simulink model "buck1"  (Simulink 6.1)
settings: Solver=ode45  StartTime=0.0  StopTime=0.01  RelTol=1e-3
libraries: powerlib x11
settings Model: Creator=USRE  LastModifiedBy=Sreejith
settings OptimizationCC: InlineInvariantSignals=off  InitFltsAndDblsToZero=off
settings DebuggingCC: SignalResolutionControl=UseLocalSettings  SolverPrmCheckMsg=warning  MultiTaskDSMMsg=error
settings GRTTargetCC: TargetFcnLib=ansi_tfl_table_tmw.mat

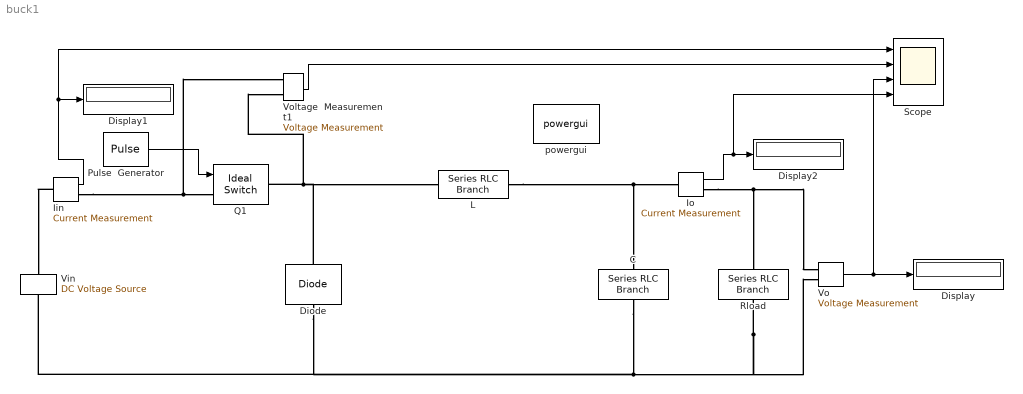
== system buck1 ==
  C : powerlib/Elements/Series RLC Branch  Orientation=down  PhysicalDomain=powersysdomain  SubClassName=unknown  LeftPortType=p1  RightPortType=p1  LConnTagsString=__new0  RConnTagsString=__new0  Resistance=0.1  Inductance=1e-3  Capacitance=120e-6  Measurements=Branch voltage
  Diode : powerlib/Power Electronics/Diode  Orientation=up  Ron=0.001  Lon=0  Vf=0.8  IC=0  Rs=500  Cs=250e-9  Measurements=off
  Display : Display
  Display1 : Display
  Display2 : Display
  Iin : powerlib/Measurements/Current Measurement  PhasorSimulation=off  OutputType=Complex  PSBequivalent=0
  Io : powerlib/Measurements/Current Measurement  PhasorSimulation=off  OutputType=Complex  PSBequivalent=0
  L : powerlib/Elements/Series RLC Branch  PhysicalDomain=powersysdomain  SubClassName=unknown  LeftPortType=p1  RightPortType=p1  LConnTagsString=__new0  RConnTagsString=__new0  Resistance=1  Inductance=11.5e-6  Capacitance=1e-6  Measurements=None
  Pulse  Generator : DiscretePulseGenerator  PulseType=Time based  Period=1/(100e3)  PulseWidth=50
  Q1 : powerlib/Power Electronics/Ideal Switch  Ron=0.001  Lon=0  IC=0  Rs=1e5  Cs=inf  Measurements=off
  Rload : powerlib/Elements/Series RLC Branch  Orientation=down  PhysicalDomain=powersysdomain  SubClassName=unknown  LeftPortType=p1  RightPortType=p1  LConnTagsString=__new0  RConnTagsString=__new0  Resistance=2  Inductance=1e-3  Capacitance=150e-6  Measurements=Branch voltage
  Scope : Scope  NumInputPorts=4
      settings: TimeRange=2.375478927332895e-010  YMin=0~0~-5~-5  YMax=3.4~3~5~5
  "Vin " : powerlib/Electrical Sources/DC Voltage Source  Orientation=up  Amplitude=12  Measurements=None
  Vo : powerlib/Measurements/Voltage Measurement  PhasorSimulation=off  OutputType=Complex  PSBequivalent=0
  Voltage  Measurement1 : powerlib/Measurements/Voltage Measurement  PhasorSimulation=off  OutputType=Complex  PSBequivalent=0
  powergui : powerlib/powergui  Priority=1  SimulationMode=Continuous  SampleTime=50e-6  echomessages=off  Frange=[0:2:500]  Ylog=off  Xlog=on  save=off  variable=ZData  ZoomFFT=on  StartTime=0.0  cycles=1  DisplayStyle=1  fundamental=60  FreqAxis=off  MaxFrequency=1000  frequencyindice=0  frequencyindicesteady=1  RmsSteady=1  display=off  Ts=0  frequency=60  methode=off
  wires:
  Vo/1 -> Display/1, Scope/3
  Io/1 -> Display2/1, Scope/4
  Iin/1 -> Display1/1, Scope/1
  Pulse  Generator/1 -> Q1/1
  Voltage  Measurement1/1 -> Scope/2
  connections:
  L/LConn1 -- Diode/RConn1 -- Q1/RConn1 -- Voltage  Measurement1/LConn2
  Iin/RConn1 -- Q1/LConn1 -- Voltage  Measurement1/LConn1
  L/RConn1 -- Io/LConn1 -- C/LConn1
  Diode/LConn1 -- "Vin "/LConn1 -- Rload/RConn1 -- Vo/LConn2 -- C/RConn1
  Iin/LConn1 -- "Vin "/RConn1
  Io/RConn1 -- Rload/LConn1 -- Vo/LConn1
